simulink model "ats"  (Simulink 8.8)
settings: Solver=VariableStepAuto  StartTime=0.0  StopTime=30  FixedStep=0.1  RelTol=1e-3  EnableMultiTasking=on
libraries: Solver_SF x1
settings Model: Creator=think  LastModifiedBy=think
settings SolverCC: AutoInsertRateTranBlk=on
settings DataIOCC: SaveFormat=Dataset  SignalLoggingSaveFormat=Dataset
settings DebuggingCC: UnderspecifiedInitializationDetection=Simplified  MergeDetectMultiDrivingBlocksExec=error  FcnCallInpInsideContextMsg=error  AllowSymbolicDim=off  StateNameClashWarn=none
settings HardwareCC: ProdBitPerPointer=64  ProdBitPerSizeT=64  ProdBitPerPtrDiffT=64  ProdLargestAtomicFloat=Float  ProdIntDivRoundTo=Zero  ProdEndianess=LittleEndian  ProdWordSize=64  ProdHWDeviceType=Intel->x86-64 (Windows64)
settings ModelReferenceCC: PropagateSignalLabelsOutOfModel=on
settings GRTTargetCC: CombineOutputUpdateFcns=on  GRTInterface=off
settings ConfigComp: CovSFcnEnable=off

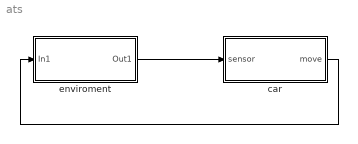
== system ats ==
  car : Subsystem
  enviroment : Subsystem
  wires:
  enviroment/1(Out1) -> car/1(sensor)
  car/1(move) -> enviroment/1(In1)

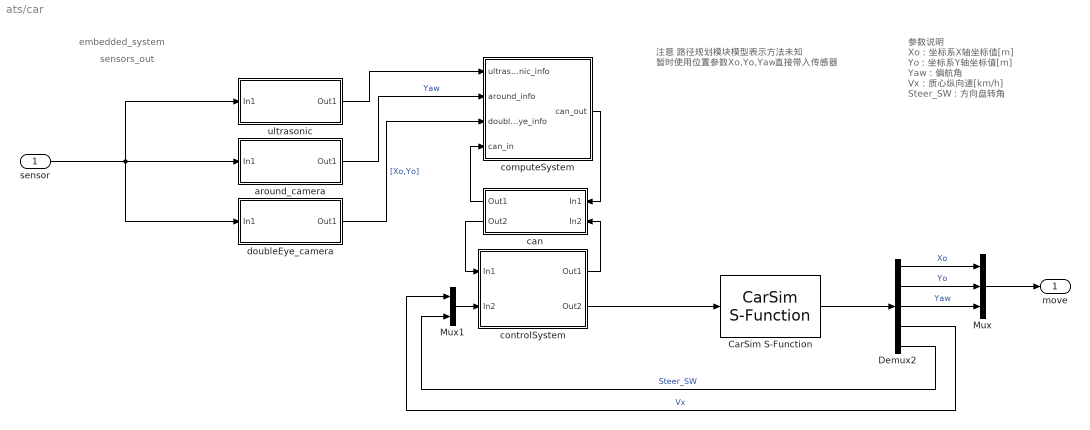
== system ats/car ==
  note: 注意
      | 路径规划模块模型表示方法未知
      | 暂时使用位置参数Xo,Yo,Yaw直接带入传感器
  note: 参数说明
      | Xo：坐标系X轴坐标值[m]
      | Yo：坐标系Y轴坐标值[m]
      | Yaw：偏航角
      | Vx：质心纵向速[km/h]
      | Steer_SW：方向盘转角
  note: embedded_system
  note: sensors_out
  sensor : Inport
  CarSim S-Function : Solver_SF/CarSim S-Function  Priority=1  VehicleCode=i_i  SIMFILE=simfile
  Demux2 : Demux  Outputs=5
  Mux : Mux  Inputs=3
  Mux1 : Mux  Inputs=2
  around_camera : Subsystem
  can : Subsystem
  computeSystem : Subsystem
  controlSystem : Subsystem
  doubleEye_camera : Subsystem
  ultrasonic : Subsystem
  move : Outport
  wires:
  sensor/1 -> doubleEye_camera/1(In1), ultrasonic/1(In1), around_camera/1(In1)
  computeSystem/1(can_out) -> can/1(In1)
  can/1(Out1) -> computeSystem/4(can_in)
  can/2(Out2) -> controlSystem/1(In1)
  ultrasonic/1(Out1) -> computeSystem/1(ultrasonic_info)
  around_camera/1(Out1) -> computeSystem/2(around_info)  "Yaw"
  doubleEye_camera/1(Out1) -> computeSystem/3(doubleEye_info)  "[Xo,Yo]"
  controlSystem/2(Out2) -> CarSim S-Function/1
  CarSim S-Function/1 -> Demux2/1
  Demux2/5 -> Mux1/2  "Steer_SW"
  Demux2/4 -> Mux1/1  "Vx"
  Demux2/1 -> Mux/1  "Xo"
  controlSystem/1(Out1) -> can/2(In2)
  Demux2/2 -> Mux/2  "Yo"
  Demux2/3 -> Mux/3  "Yaw"
  Mux/1 -> move/1
  Mux1/1 -> controlSystem/2(In2)

== system ats/enviroment ==
  In1 : Inport
  Out1 : Outport
  wires:
  In1/1 -> Out1/1

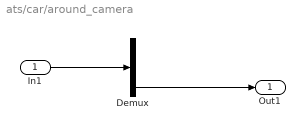
== system ats/car/around_camera ==
  In1 : Inport
  Demux : Demux  Outputs=3
  Out1 : Outport
  wires:
  In1/1 -> Demux/1
  Demux/3 -> Out1/1

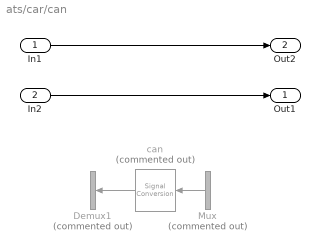
== system ats/car/can ==
  In1 : Inport
  In2 : Inport  Port=2
  Demux1 : Demux  Commented=on  Outputs=2
  Mux : Mux  Commented=on  Inputs=2
  can : SignalConversion  Commented=on  ConversionOutput=Nonvirtual bus  OutDataTypeStr=Bus: can  OverrideOpt=off
  Out1 : Outport
  Out2 : Outport  Port=2
  wires:
  Mux/1 -> can/1
  can/1 -> Demux1/1
  In1/1 -> Out2/1
  In2/1 -> Out1/1

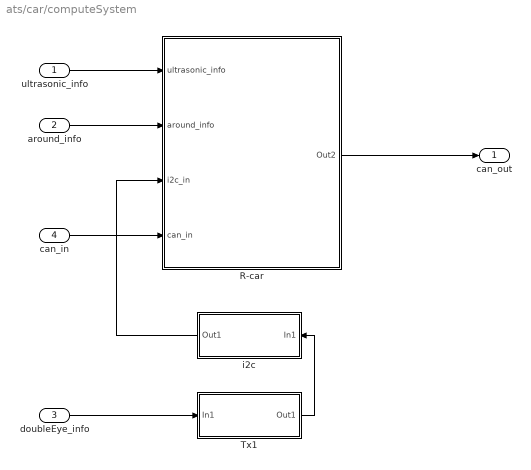
== system ats/car/computeSystem ==
  ultrasonic_info : Inport
  around_info : Inport  Port=2
  doubleEye_info : Inport  Port=3
  can_in : Inport  Port=4
  R-car : Subsystem
  Tx1 : Subsystem
  i2c : Subsystem
  can_out : Outport
  wires:
  ultrasonic_info/1 -> R-car/1(ultrasonic_info)
  doubleEye_info/1 -> Tx1/1(In1)
  around_info/1 -> R-car/2(around_info)
  Tx1/1(Out1) -> i2c/1(In1)
  i2c/1(Out1) -> R-car/3(i2c_in)
  R-car/1(Out2) -> can_out/1
  can_in/1 -> R-car/4(can_in)

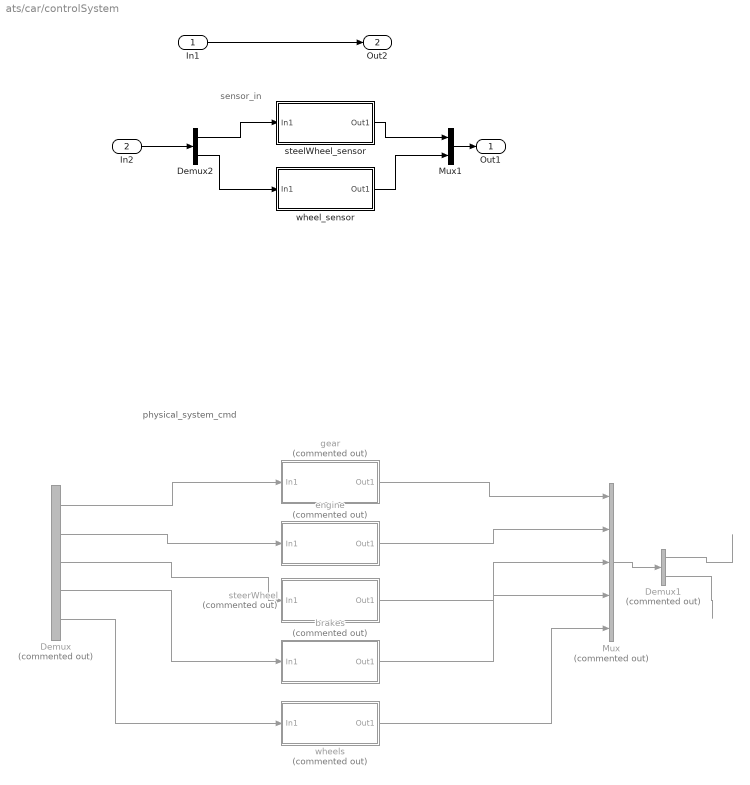
== system ats/car/controlSystem ==
  note: physical_system_cmd
  note: sensor_in
  In1 : Inport
  In2 : Inport  Port=2
  Demux : Demux  Commented=on  Outputs=5
  Demux1 : Demux  Commented=on  Outputs=2
  Demux2 : Demux  Outputs=2
  Mux : Mux  Commented=on  Inputs=5
  Mux1 : Mux  Inputs=2
  brakes : Subsystem  Commented=on
  engine : Subsystem  Commented=on
  gear : Subsystem  Commented=on
  steelWheel_sensor : Subsystem
  steerWheel : Subsystem  Commented=on
  wheel_sensor : Subsystem
  "wheels " : Subsystem  Commented=on
  Out1 : Outport
  Out2 : Outport  Port=2
  wires:
  Demux/1 -> gear/1(In1)
  Demux/2 -> engine/1(In1)
  Demux/3 -> steerWheel/1(In1)
  Demux/4 -> brakes/1(In1)
  Demux/5 -> "wheels "/1(In1)
  gear/1(Out1) -> Mux/1
  engine/1(Out1) -> Mux/2
  steerWheel/1(Out1) -> Mux/3
  brakes/1(Out1) -> Mux/4
  "wheels "/1(Out1) -> Mux/5
  Mux/1 -> Demux1/1
  Demux1/1 -> ?
  Demux1/2 -> ?
  In2/1 -> Demux2/1
  Demux2/2 -> wheel_sensor/1(In1)
  Demux2/1 -> steelWheel_sensor/1(In1)
  wheel_sensor/1(Out1) -> Mux1/2
  steelWheel_sensor/1(Out1) -> Mux1/1
  Mux1/1 -> Out1/1
  In1/1 -> Out2/1

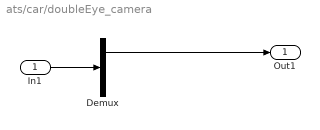
== system ats/car/doubleEye_camera ==
  In1 : Inport
  Demux : Demux  Outputs=[2,1]
  Out1 : Outport
  wires:
  In1/1 -> Demux/1
  Demux/1 -> Out1/1

== system ats/car/ultrasonic ==
  In1 : Inport
  Out1 : Outport
  wires:
  In1/1 -> Out1/1

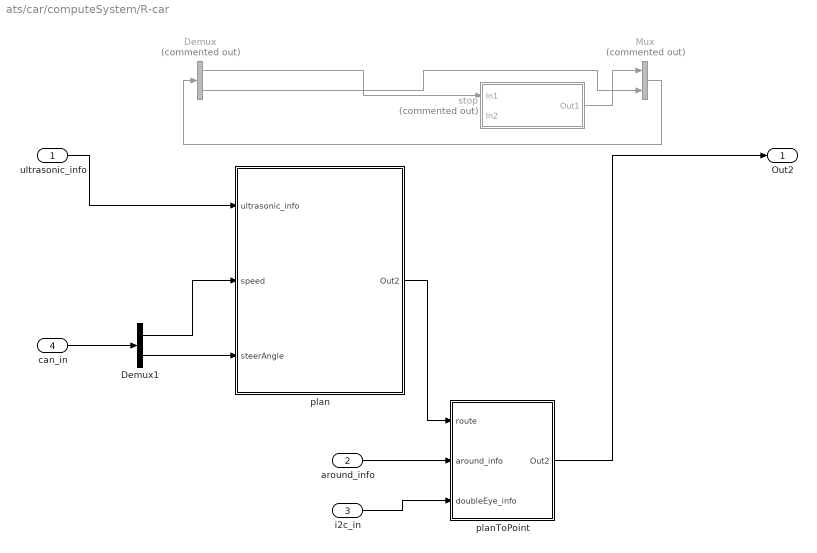
== system ats/car/computeSystem/R-car ==
  ultrasonic_info : Inport
  around_info : Inport  Port=2
  i2c_in : Inport  Port=3
  can_in : Inport  Port=4
  Demux : Demux  Commented=on  Outputs=2
  Demux1 : Demux  Outputs=2
  Mux : Mux  Commented=on  Inputs=2
  plan : Subsystem
  planToPoint : Subsystem
  stop : Subsystem  Commented=on
  Out2 : Outport
  wires:
  ultrasonic_info/1 -> plan/1(ultrasonic_info)
  plan/1(Out2) -> planToPoint/1(route)
  around_info/1 -> planToPoint/2(around_info)
  Demux/2 -> Mux/2
  Demux/1 -> stop/1(In1)
  Mux/1 -> Demux/1
  planToPoint/1(Out2) -> Out2/1
  can_in/1 -> Demux1/1
  Demux1/1 -> plan/2(speed)
  Demux1/2 -> plan/3(steerAngle)
  stop/1(Out1) -> Mux/1
  i2c_in/1 -> planToPoint/3(doubleEye_info)

== system ats/car/computeSystem/Tx1 ==
  In1 : Inport
  Chart : Stateflow chart  Commented=on  TreatAsAtomicUnit=on
  Out1 : Outport
  wires:
  In1/1 -> Out1/1

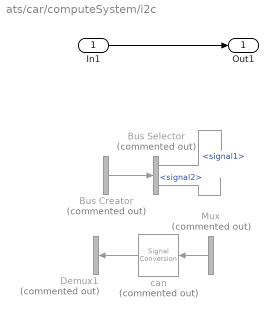
== system ats/car/computeSystem/i2c ==
  In1 : Inport
  Bus Creator : BusCreator  Commented=on  Inputs=2
  Bus Selector : BusSelector  Commented=on  OutputSignals=signal1,signal2
  Demux1 : Demux  Commented=on  Outputs=2
  Mux : Mux  Commented=on  Inputs=2
  can : SignalConversion  Commented=on  ConversionOutput=Nonvirtual bus  OutDataTypeStr=Bus: can  OverrideOpt=off
  Out1 : Outport
  wires:
  In1/1 -> Out1/1
  Mux/1 -> can/1
  can/1 -> Demux1/1
  Bus Selector/1 -> ?  "<signal1>"
  Bus Selector/2 -> ?  "<signal2>"
  Bus Creator/1 -> Bus Selector/1

== system ats/car/controlSystem/brakes ==
  In1 : Inport
  Out1 : Outport
  wires:
  In1/1 -> Out1/1

== system ats/car/controlSystem/engine ==
  In1 : Inport
  Out1 : Outport
  wires:
  In1/1 -> Out1/1

== system ats/car/controlSystem/gear ==
  In1 : Inport
  Out1 : Outport
  wires:
  In1/1 -> Out1/1

== system ats/car/controlSystem/steelWheel_sensor ==
  In1 : Inport
  Out1 : Outport
  wires:
  In1/1 -> Out1/1

== system ats/car/controlSystem/steerWheel ==
  In1 : Inport
  Out1 : Outport
  wires:
  In1/1 -> Out1/1

== system ats/car/controlSystem/wheel_sensor ==
  In1 : Inport
  Out1 : Outport
  wires:
  In1/1 -> Out1/1

== system ats/car/controlSystem/wheels  ==
  In1 : Inport
  Out1 : Outport
  wires:
  In1/1 -> Out1/1

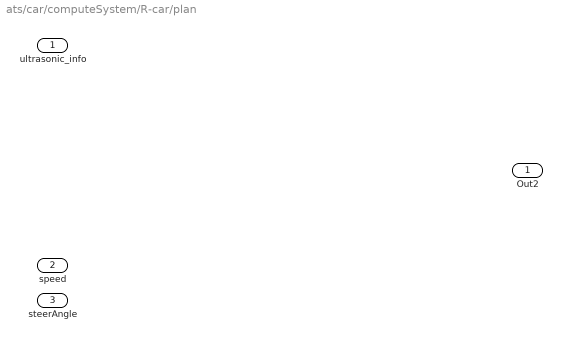
== system ats/car/computeSystem/R-car/plan ==
  ultrasonic_info : Inport
  speed : Inport  Port=2
  steerAngle : Inport  Port=3
  Out2 : Outport

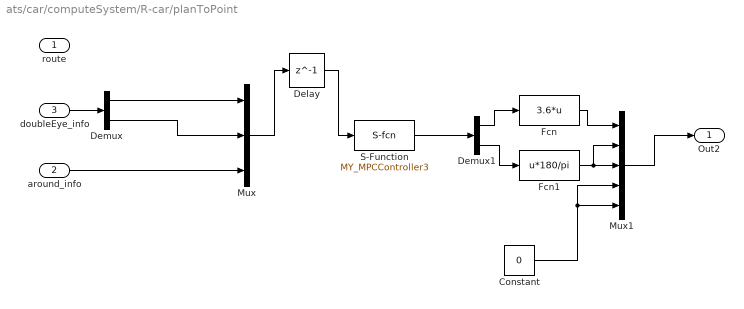
== system ats/car/computeSystem/R-car/planToPoint ==
  route : Inport
  around_info : Inport  Port=2
  doubleEye_info : Inport  Port=3
  Constant : Constant  Value=0
  Delay : Delay  DelayLength=1  InitialCondition=0
  Demux : Demux  Outputs=2
  Demux1 : Demux  Outputs=2
  Fcn : Fcn  Expr=3.6*u
  Fcn1 : Fcn  Expr=u*180/pi
  Mux : Mux  Inputs=3
  Mux1 : Mux  Inputs=5
  S-Function : S-Function  FunctionName=MY_MPCController3  SFunctionDeploymentMode=off  EnableBusSupport=off
  Out2 : Outport
  wires:
  Mux/1 -> Delay/1
  doubleEye_info/1 -> Demux/1
  S-Function/1 -> Demux1/1
  Demux/1 -> Mux/1
  Demux/2 -> Mux/2
  around_info/1 -> Mux/3
  Mux1/1 -> Out2/1
  Fcn/1 -> Mux1/1
  Fcn1/1 -> Mux1/3, Mux1/2
  Demux1/1 -> Fcn/1
  Demux1/2 -> Fcn1/1
  Constant/1 -> Mux1/4, Mux1/5
  Delay/1 -> S-Function/1

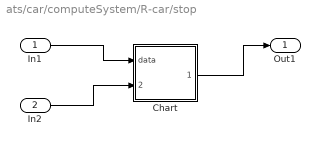
== system ats/car/computeSystem/R-car/stop ==
  In1 : Inport
  In2 : Inport  Port=2
  Chart : Stateflow chart  TreatAsAtomicUnit=on
  Out1 : Outport
  wires:
  In1/1 -> Chart/1(data)
  In2/1 -> Chart/2(data2)
  Chart/1(data1) -> Out1/1

== stateflow chart car/computeSystem/Tx1/Chart ==
  data: data input double; data1 output double

== stateflow chart car/computeSystem/R-car/stop/Chart ==
  data: data input double; data1 output double; data2 input double
